simulink model "Test_Program_Counter"  (Simulink 8.1)
settings: Solver=ode45  StartTime=0.0  StopTime=20.0  RelTol=1e-3
undefined symbols (not defined in the file): sigbuilder_block
libraries: simulink_extras x1, Computer_Library x1
settings Model: Creator=uzivatel  LastModifiedBy=uzivatel
settings DataIOCC: SignalLoggingSaveFormat=Dataset
settings OptimizationCC: ExpressionDepthLimit=128
settings DebuggingCC: FcnCallInpInsideContextMsg=EnableAllAsError
settings GRTTargetCC: CombineOutputUpdateFcns=on  GRTInterface=off

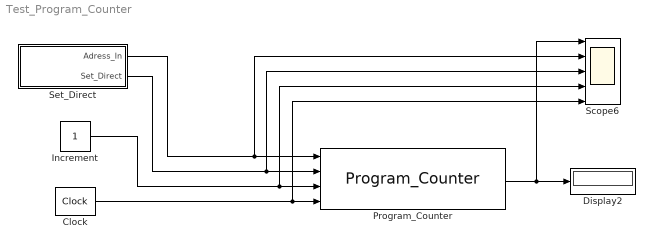
== system Test_Program_Counter ==
  Clock : simulink_extras/Flip Flops/Clock  period=1
  Display2 : Display
  Increment : Constant  OutDataTypeStr=boolean
  Program_Counter : Computer_Library/Program_Counter
  Scope6 : Scope  NumInputPorts=5
      settings: YMin=0~0~0~0~0  YMax=20~20~1.5~1.5~1.5
  Set_Direct : Subsystem  Tag=STV Subsys  LoadFcn=sigbuilder_block('load',[51.75 6 549.75 321 ]);  StartFcn=sigbuilder_block('start');  StopFcn=sigbuilder_block('stop');  ClipboardFcn=sigbuilder_block('clipboard');  mask(Sigbuilder block){}
      mask help: Simulink:masks:SigbuilderBlock_MD
      mask init:
      | if ~strcmp(get_param(bdroot(gcbh),'SimulationStatus'),'stopped') tuvar = sigbuilder_block('maskInit'); end
      settings: CopyFcn=sigbuilder_block('copy');  DeleteFcn=sigbuilder_block('delete');  ModelCloseFcn=sigbuilder_block('modelClose');  PreSaveFcn=sigbuilder_block('preSave');  PauseFcn=sigbuilder_block('pause');  ContinueFcn=sigbuilder_block('continue');  NameChangeFcn=sigbuilder_block('namechange');  OpenFcn=sigbuilder_block('open',[51.75 6 549.75 321 ]);  CloseFcn=sigbuilder_block('close');
      mask Display: plot(0, 0, 100, 100,[2, 2, 32, 32, 2], [68, 8, 8, 68, 68],[32, 2], [38, 38], [32, 19, 2],[53, 60, 44], [32, 17, 17, 2],[16, 16, 31, 31]);txt = getActiveGroup(gcbh);text(2, 100, txt,'verticalAlignment', 'top');
  wires:
  Increment/1 -> Scope6/4, Program_Counter/3
  Set_Direct/2(Set_Direct) -> Program_Counter/2, Scope6/3
  Set_Direct/1(Adress_In) -> Scope6/2, Program_Counter/1
  Clock/1 -> Scope6/5, Program_Counter/4
  Program_Counter/1 -> Display2/1, Scope6/1

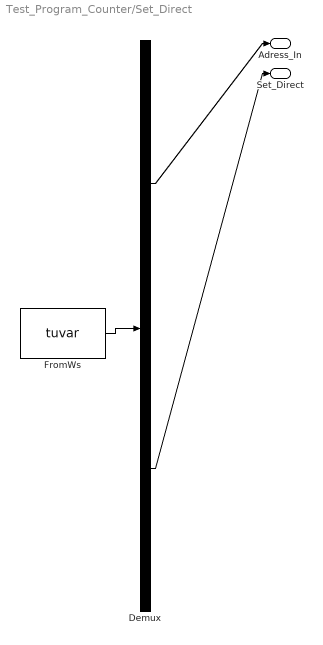
== system Test_Program_Counter/Set_Direct ==
  Demux : Demux  Tag=STV Demux  Outputs=2
  FromWs : FromWorkspace  Tag=STV FromWs  VariableName=tuvar  SampleTime=0  SigBuilderData=DataTag0  VnvData=DataTag1
      SigBuilderData=|
      | common.afterFinalStr = 'Extrapolate'
      | common.sampleTime = 0
      | dataSet.timeRange = [0 20]
      | dataSet.name = 'Group 1'
      | sbobj.Groups.Name = 'Group 1'
      | sbobj.Groups.Signals(1).Name = 'Adress_In'
      | sbobj.Groups.Signals(1).XData = [0 1 1 2 2 8 8 9 9 20]
      | sbobj.Groups.Signals(1).YData = [0 0 14 14 0 0 13 13 0 0]
      | sbobj.Groups.Signals(2).Name = 'Set_Direct'
      | sbobj.Groups.Signals(2).XData = [0 1 1 2 2 8 8 9 9 20]
      | sbobj.Groups.Signals(2).YData = [0 0 1 1 0 0 1 1 0 0]
      | sbobj.Groups.TimeRange = [0 20]
  Adress_In : Outport  Tag=STV Outport
  Set_Direct : Outport  Tag=STV Outport  Port=2
  wires:
  FromWs/1 -> Demux/1
  Demux/1 -> Adress_In/1
  Demux/2 -> Set_Direct/1
